simulink model "exercise7"  (R2017a)
settings: Solver=VariableStepAuto  StartTime=0.0  StopTime=30  RelTol=1e-3
settings Model: Creator=viktor  LastModifiedBy=viktor

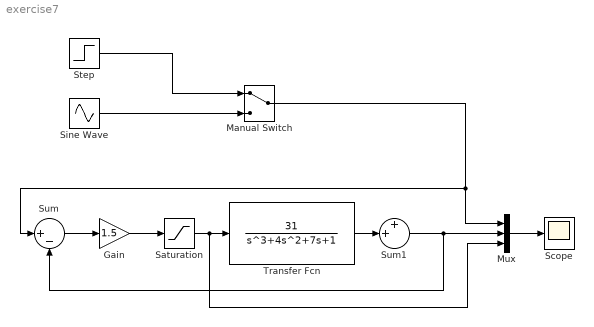
== system exercise7 ==
  Gain : Gain  Gain=1.5
  Manual Switch : ManualSwitch
  Mux : Mux  Inputs=3
  Saturation : Saturate  UpperLimit=3  LowerLimit=-3
  Scope : Scope
  Sine Wave : Sin  Amplitude=.01  Frequency=3  SampleTime=0
  Step : Step  Before=0.1  After=0  SampleTime=0
  Sum : Sum  Inputs=|+-
  Sum1 : Sum  Inputs=++|
  Transfer Fcn : TransferFcn  Numerator=[31]  Denominator=[1 4 7 1]
  wires:
  Gain/1 -> Saturation/1
  Saturation/1 -> Mux/3, Transfer Fcn/1
  Sum/1 -> Gain/1
  Mux/1 -> Scope/1
  Transfer Fcn/1 -> Sum1/2
  Sum1/1 -> Sum/2, Mux/2
  Sine Wave/1 -> Manual Switch/2
  Step/1 -> Manual Switch/1
  Manual Switch/1 -> Mux/1, Sum/1
